simulink model "NMPCexp"  (R2019b)
settings: Solver=ode1  StartTime=0.0  StopTime=inf  FixedStep=Ts  RelTol=1e-3  EnableMultiTasking=on
PostLoadFcn:
  | qc_set_target_type(getConfigSet(bdroot, 'QUARC Default Target Configuration'));
values from neighbouring files (symbols this model uses):
  Parameters = [bm,g,I2,Jeq,Jm,Kf1,Kf2,Km,Ks,l1,l2,m1,m2,Rm,x1,x2]    [NMPCswingup.m]
  Ts = 0.1    [NMPCswingup.m]    (also in PendulumStateFcn.m = u(2))
  yref = [1.5 pi]    [NMPCswingup.m]
undefined symbols (not defined in the file or in its folder): HIL, qc_get_step_size
libraries: quarc_library x4, mpclib x1
settings Model: SimulationMode=external  ExtModeTrigDuration=5000  Creator=CFulford  LastModifiedBy=Student
settings SolverCC: PositivePriorityOrder=on
settings DataIOCC: LimitDataPoints=on  SaveFormat=Array  SignalLoggingSaveFormat=ModelDataLogs  ReturnWorkspaceOutputs=off
settings OptimizationCC: ExpressionDepthLimit=2147483647  InitFltsAndDblsToZero=on  LifeSpan=inf
settings DebuggingCC: SaveWithParameterizedLinksMsg=none  UnderspecifiedInitializationDetection=Classic  MergeDetectMultiDrivingBlocksExec=none  SolverPrmCheckMsg=warning  MultiTaskDSMMsg=warning  MultiTaskCondExecSysMsg=none  FcnCallInpInsideContextMsg=warning  StateNameClashWarn=warning  SFUnexpectedBacktrackingDiag=warning  SFNoUnconditionalDefaultTransitionDiag=warning  SFExecutionAtInitializationDiag=none  ArithmeticOperatorsInVariantConditions=warning
settings HardwareCC: ProdBitPerPointer=32  ProdBitPerSizeT=32  ProdBitPerPtrDiffT=32  ProdLargestAtomicFloat=None  ProdIntDivRoundTo=Undefined  ProdEndianess=Unspecified  ProdWordSize=32  ProdHWDeviceType=32-bit Generic
settings ModelReferenceCC: PropagateSignalLabelsOutOfModel=off
settings SFSimCC: SimUseLocalCustomCode=off  CustomCodeUndefinedFunction=UseInterfaceOnly
settings RTWCC: Description=QUARC Win64 Target  SystemTargetFile=quarc_win64.tlc  TemplateMakefile=quarc_default_tmf  RTWUseLocalCustomCode=off
settings CodeAppCC: StateflowObjectComments=on
settings STFCustomTargetCC: TargetPreCompLibLocation=C:\PROGRA~3\QUARC\lib\2019b\win64\release  ConcurrentExecutionCompliant=on  GeneratePreprocessorConditionals=Disable all  CombineOutputUpdateFcns=on  CPPClassGenCompliant=on  SystemTargetFile=quarc_win64.tlc
settings GRTTargetCC: TargetPreCompLibLocation=C:\PROGRA~3\QUARC\lib\2019b\win64\release  TargetLangStandard=C89/C90 (ANSI)  ParMdlRefBuildCompliant=off  CompOptLevelCompliant=off  GeneratePreprocessorConditionals=Disable all  MatFileLogging=off  UseToolchainInfoCompliant=off  ExtMode=on  ExtModeMexFile=quarc_comm
settings ConfigComp: CovMetricSettings=dw  CovHtmlReporting=on  CovSaveCumulativeToWorkspaceVar=on  CovSaveSingleToWorkspaceVar=on  CovExternalEMLEnable=off  CovSFcnEnable=off

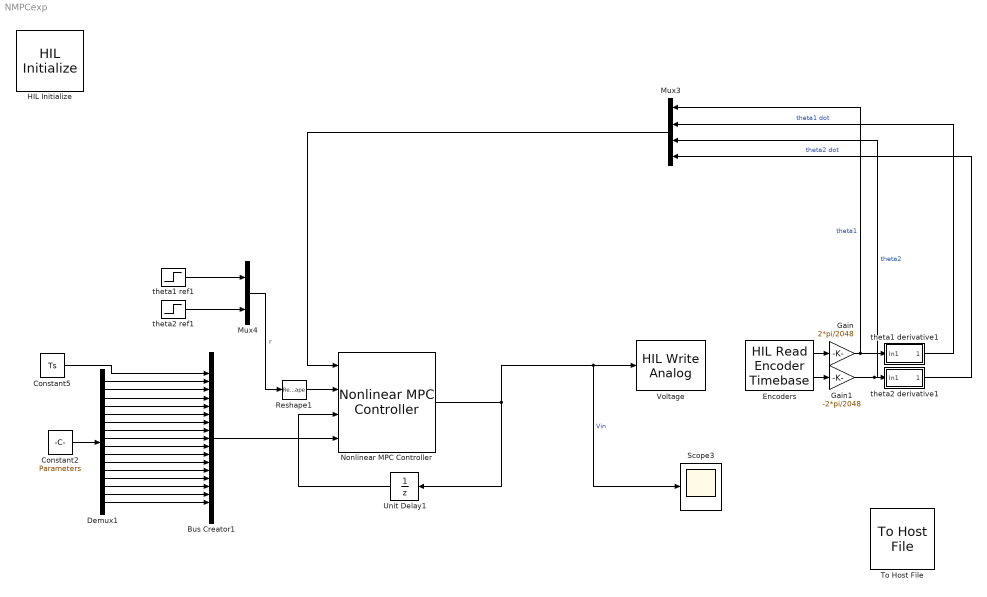
== system NMPCexp ==
  Bus Creator1 : BusCreator  Inputs=17  OutDataTypeStr=Bus: customBusObject  NonVirtualBus=on
  Constant2 : Constant  Value=Parameters
  Constant5 : Constant  Value=Ts
  Demux1 : Demux  Outputs=16
  Encoders : quarc_library/Data Acquisition/Generic/Timebases/HIL Read Encoder Timebase  object_name=HIL-1  clock=0  channels=[0:1]  samples_in_buffer=max(ceil(1/qc_get_step_size), 1)  active=on  vector_output=off  data_type_mode=Inherit via back propagation  data_type=double
  Gain : Gain  Gain=2*pi/2048
  Gain1 : Gain  Gain=-2*pi/2048
  HIL Initialize : quarc_library/Data Acquisition/Generic/Configuration/HIL Initialize  Priority=-99  object_name=HIL-1  board_type=qube_servo2_usb  board_number=0  board_options=""  exclusive=off  active=off  hardware_clocks=[0]  clock_modes=[]  initial_clock_frequencies=[]  set_clock_params_at_start=off  set_clock_params_at_switch_in=off  set_clock_frequencies_at_start=off  set_clock_frequencies_at_switch_in=off  analog_input_channels=[0]  analog_input_configurations=[]  analog_input_maximums=3  analog_input_minimums=-3  set_analog_input_params_at_start=off  set_analog_input_params_at_switch_in=off  analog_output_channels=[0]  analog_output_maximums=15  analog_output_minimums=-15  initial_analog_outputs=[0]  final_analog_outputs=[0]  watchdog_analog_outputs=0  set_analog_output_params_at_start=off  set_analog_output_params_at_switch_in=off  set_analog_outputs_at_start=on  set_analog_outputs_at_switch_in=off  set_analog_outputs_at_terminate=on  set_analog_outputs_at_switch_out=off  set_analog_outputs_on_watchdog=on  digital_input_channels=[]  digital_output_channels=[0]  digital_output_configuration=[]  initial_digital_outputs=[1]  final_digital_outputs=[0]  watchdog_digital_outputs=[0]  set_digital_output_params_at_start=off  set_digital_output_params_at_switch_in=off  set_digital_outputs_at_start=on  set_digital_outputs_at_switch_in=off  set_digital_outputs_at_terminate=on  set_digital_outputs_at_switch_out=off  set_digital_outputs_on_watchdog=on  encoder_channels=[0:1]  quadrature=[4]  encoder_filter_frequency=[]  initial_encoder_counts=[0]  set_encoder_params_at_start=off  set_encoder_params_at_switch_in=off  set_encoder_counts_at_start=on  set_encoder_counts_at_switch_in=off  pwm_channels=[]  pwm_modes=[]  pwm_frequency=[]  pwm_configuration=[]  pwm_alignment=[]  pwm_polarity=[]  pwm_leading_deadband=[]  pwm_trailing_deadband=[]  initial_pwm_outputs=[]  final_pwm_outputs=[]  watchdog_pwm_outputs=[]  set_pwm_params_at_start=off  set_pwm_params_at_switch_in=off  set_pwm_outputs_at_start=off  set_pwm_outputs_at_switch_in=off  set_pwm_outputs_at_terminate=off  set_pwm_outputs_at_switch_out=off  set_pwm_outputs_on_watchdog=off  other_output_channels=[11000:11002]  initial_other_outputs=[0 1 0]  final_other_outputs=[1 0 0]  watchdog_other_outputs=[0 0 1]  set_other_outputs_at_start=on  set_other_outputs_at_switch_in=off  set_other_outputs_at_terminate=on  set_other_outputs_at_switch_out=off  set_other_outputs_on_watchdog=on
  Mux3 : Mux
  Mux4 : Mux  Inputs=2
  Nonlinear MPC Controller : mpclib/Nonlinear MPC Controller  nlmpcobj=nlobj  UseObjectTs=on  TsControl=Ts  md_enabled=off  mvtarget_enabled=off  param_enabled=on  cost_enabled=off  mvseq_enabled=off  stateseq_enabled=off  ovseq_enabled=off  slack_enabled=off  status_enabled=off  ov_min=off  ov_max=off  mv_min=off  mv_max=off  mvrate_min=off  mvrate_max=off  state_min=off  state_max=off  ov_weight=off  mv_weight=off  mvrate_weight=off  ecr_weight=off  nlp_initialize=off
      settings: SourceProductName=Model Predictive Control Toolbox
  Reshape1 : Reshape  OutputDimensionality=Row vector (2-D)
  Scope3 : Scope
  To Host File : quarc_library/Sinks/To Host/To Host File  file_name=data_%{date}_%{time}.mat  variable_name=data_%{date}_%{time}  decimation=1  sample_time=-1  file_format=MAT-file v.5  options=No header or footer  append=off  final_file_name=data_28-May-2024_17-01-25.mat  bitrate=2000000
  Unit Delay1 : UnitDelay  SampleTime=-1  HasFrameUpgradeWarning=on
  Voltage : quarc_library/Data Acquisition/Generic/Immediate I//O/HIL Write Analog  object_name=HIL-1  channels=0  sample_time=-1  active=off  vector_input=off
  theta1 derivative1 : Subsystem
  theta1 ref1 : Step  Time=10  After=yref(1)  SampleTime=0
  theta2 derivative1 : Subsystem
  theta2 ref1 : Step  Time=0  After=yref(2)  SampleTime=0
  wires:
  Demux1/9 -> Bus Creator1/10
  Demux1/5 -> Bus Creator1/6
  Demux1/1 -> Bus Creator1/2
  Nonlinear MPC Controller/1 -> Voltage/1, Scope3/1, Unit Delay1/1  "Vin"
  Bus Creator1/1 -> Nonlinear MPC Controller/4
  Demux1/6 -> Bus Creator1/7
  Demux1/13 -> Bus Creator1/14
  Demux1/11 -> Bus Creator1/12
  Demux1/12 -> Bus Creator1/13
  Demux1/8 -> Bus Creator1/9
  theta1 ref1/1 -> Mux4/1
  Demux1/10 -> Bus Creator1/11
  Demux1/14 -> Bus Creator1/15
  Demux1/7 -> Bus Creator1/8
  Demux1/15 -> Bus Creator1/16
  Constant2/1 -> Demux1/1
  Unit Delay1/1 -> Nonlinear MPC Controller/3
  Demux1/2 -> Bus Creator1/3
  Mux4/1 -> Reshape1/1  "r"
  Demux1/16 -> Bus Creator1/17
  Reshape1/1 -> Nonlinear MPC Controller/2
  Constant5/1 -> Bus Creator1/1
  Demux1/3 -> Bus Creator1/4
  Demux1/4 -> Bus Creator1/5
  theta2 ref1/1 -> Mux4/2
  Encoders/1 -> Gain/1
  Encoders/2 -> Gain1/1
  Gain/1 -> theta1 derivative1/1(In1), Mux3/1  "theta1"
  Gain1/1 -> theta2 derivative1/1(In1), Mux3/3  "theta2"
  theta1 derivative1/1(Out1) -> Mux3/2  "theta1 dot"
  theta2 derivative1/1(Out1) -> Mux3/4  "theta2 dot"
  Mux3/1 -> Nonlinear MPC Controller/1

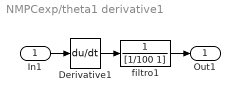
== system NMPCexp/theta1 derivative1 ==
  In1 : Inport
  Derivative1 : Derivative
  "filtro1 " : TransferFcn  Denominator=[1/100 1]
  Out1 : Outport
  wires:
  Derivative1/1 -> "filtro1 "/1
  In1/1 -> Derivative1/1
  "filtro1 "/1 -> Out1/1

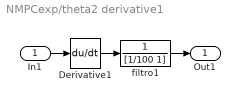
== system NMPCexp/theta2 derivative1 ==
  In1 : Inport
  Derivative1 : Derivative
  "filtro1 " : TransferFcn  Denominator=[1/100 1]
  Out1 : Outport
  wires:
  Derivative1/1 -> "filtro1 "/1
  In1/1 -> Derivative1/1
  "filtro1 "/1 -> Out1/1
